simulink model "MPC_adaptive"  (R2020b)
settings: Solver=VariableStepAuto  StartTime=0.0  StopTime=10.0  RelTol=1e-3
values from neighbouring files (symbols this model uses):
  I_mat = [I_xx I_xy I_xz ... (first row only)    [AngularDynamics_VV.m]    (also in angular_tune_test.m; temp.m)
libraries: mpclib x1, cstblocks x1
settings Model: Creator=Jonathan van Zyl  LastModifiedBy=Jonathan van Zyl

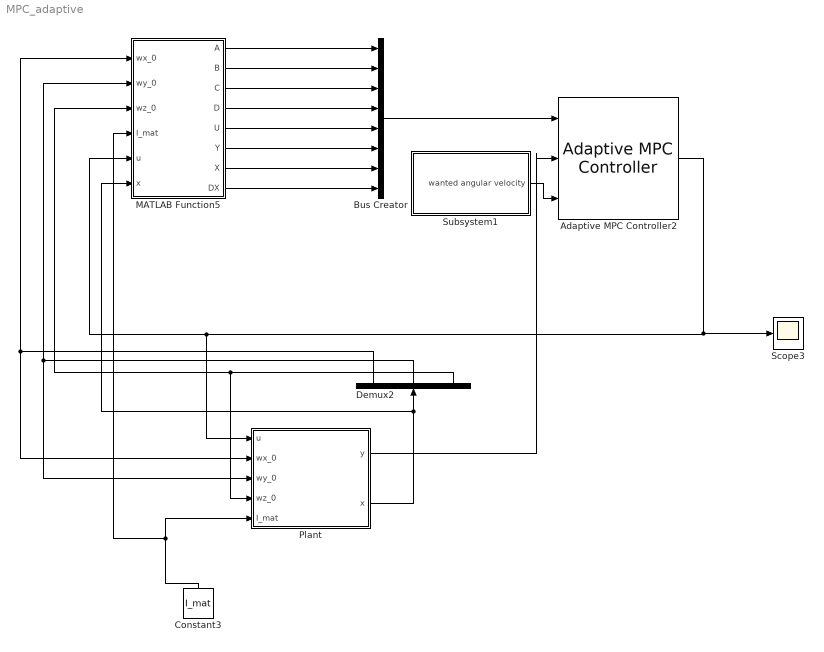
== system MPC_adaptive ==
  Adaptive MPC Controller2 : mpclib/Adaptive MPC Controller  SCDEnableBlockLinearizationSpecification=on  mpcobj=mpc1  enable_value=0  updateMPCinCallerWorkspace=on  md_inport=off  mv_inport=off  uref_inport=off  return_cost=off  return_mvseq=off  return_qpstatus=off  return_xseq=off  return_state=off  return_ovseq=off  state_inport=off  isltv_plant=off  umin_inport=off  umax_inport=off  ymin_inport=off  ymax_inport=off  cc_inport=off  ywt_inport=off  uwt_inport=off  duwt_inport=off  rhoeps_inport=off  pm_inport=off  MaximumP=10  HorizonChoice=FixedHorizon  BlockDataType=double  SampleTimeInherited=off  switch_inport=off
  Bus Creator : BusCreator  Inputs=8
  Constant3 : Constant  Value=I_mat
  Demux2 : Demux  Outputs=3
  MATLAB Function5 : MATLAB Function  TreatAsAtomicUnit=on
  Plant : Subsystem
  Scope3 : Scope
  Subsystem1 : Subsystem
  wires:
  Demux2/2 -> Plant/3(wy_0), MATLAB Function5/2(wy_0)
  Demux2/3 -> MATLAB Function5/3(wz_0), Plant/4(wz_0)
  Constant3/1 -> MATLAB Function5/4(I_mat), Plant/5(I_mat)
  MATLAB Function5/3(C) -> Bus Creator/3
  MATLAB Function5/6(Y) -> Bus Creator/6
  MATLAB Function5/2(B) -> Bus Creator/2
  MATLAB Function5/7(X) -> Bus Creator/7
  MATLAB Function5/8(DX) -> Bus Creator/8
  MATLAB Function5/1(A) -> Bus Creator/1
  MATLAB Function5/4(D) -> Bus Creator/4
  Demux2/1 -> MATLAB Function5/1(wx_0), Plant/2(wx_0)
  MATLAB Function5/5(U) -> Bus Creator/5
  Subsystem1/1(wanted angular velocity) -> Adaptive MPC Controller2/3
  Bus Creator/1 -> Adaptive MPC Controller2/1
  Plant/1(y) -> Adaptive MPC Controller2/2
  Plant/2(x) -> MATLAB Function5/6(x), Demux2/1
  Adaptive MPC Controller2/1 -> MATLAB Function5/5(u), Plant/1(u), Scope3/1

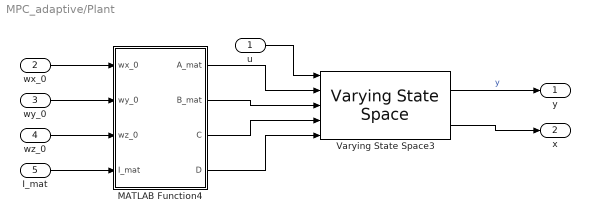
== system MPC_adaptive/Plant ==
  u : Inport
  wx_0 : Inport  Port=2
  wy_0 : Inport  Port=3
  wz_0 : Inport  Port=4
  I_mat : Inport  Port=5
  MATLAB Function4 : MATLAB Function  TreatAsAtomicUnit=on
  Varying State Space3 : cstblocks/Linear Parameter Varying/Varying State Space  x0=[0;0;0]  xNames=''  OutputX=on  OutputDX=off
  y : Outport
  x : Outport  Port=2
  wires:
  MATLAB Function4/4(D) -> Varying State Space3/5
  I_mat/1 -> MATLAB Function4/4(I_mat)
  wy_0/1 -> MATLAB Function4/2(wy_0)
  MATLAB Function4/1(A_mat) -> Varying State Space3/2
  MATLAB Function4/3(C) -> Varying State Space3/4
  wx_0/1 -> MATLAB Function4/1(wx_0)
  MATLAB Function4/2(B_mat) -> Varying State Space3/3
  Varying State Space3/1 -> y/1  "y"
  Varying State Space3/2 -> x/1
  u/1 -> Varying State Space3/1
  wz_0/1 -> MATLAB Function4/3(wz_0)

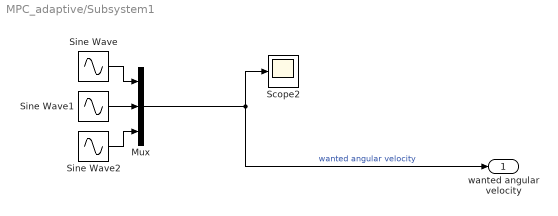
== system MPC_adaptive/Subsystem1 ==
  Mux : Mux  Inputs=3
  Scope2 : Scope
  Sine Wave : Sin  SampleTime=0
  Sine Wave1 : Sin  Amplitude=0.5  Frequency=0.7  SampleTime=0
  Sine Wave2 : Sin  Amplitude=4  Frequency=0.5  SampleTime=0
  wanted angular velocity : Outport
  wires:
  Mux/1 -> wanted angular velocity/1, Scope2/1  "wanted angular velocity"
  Sine Wave2/1 -> Mux/3
  Sine Wave/1 -> Mux/1
  Sine Wave1/1 -> Mux/2

== matlab function MPC_adaptive/Plant/MATLAB Function4 ==
  data: wx_0 input; A_mat output; wy_0 input; wz_0 input; I_mat input; B_mat output; C output; D output
function[A_mat, B_mat, C, D] = func(wx_0, wy_0, wz_0, I_mat)
I_xx = I_mat(1,1);
I_xy = I_mat(1,2);
I_xz = I_mat(1,3);

I_yx = I_mat(2,1);
I_yy = I_mat(2,2);
I_yz = I_mat(2,3);

I_zx = I_mat(3,1);
I_zy = I_mat(3,2);
I_zz = I_mat(3,3);
%% Calculate A matrix
%Calculate numerators
a = (I_yy*I_zz - I_yz*I_zy)*(I_zx*wy_0 - I_yx*wz_0) + (I_xx*I_zy - I_xy*I_zz)*(I_xx*wz_0 - I_zx*wy_0 - I_zz*wz_0) + (I_xy*I_yz - I_xz*I_yy)*(I_zx*wx_0 + I_zy*wy_0 + I_zz*wz_0 - I_yx*wy_0);
b = (I_yy*I_zz - I_yz*I_zy)*(I_zx*wx_0 + I_zy*wy_0 + I_zz*wz_0 - I_yy*wz_0) + (I_xz*I_zy - I_xy*I_zz)*(I_xy*wz_0 - I_zz*wx_0) + (I_xy*I_yz - I_xz*I_yy)*(I_zz*wx_0 - I_yx*wx_0 - I_yy*wy_0 - I_yz*wz_0);
c = (I_yy*I_zz - I_yz*I_zy)*(I_zz*wy_0 - I_yx*wx_0 - I_yy*wy_0 - I_yz*wz_0) + (I_xz*I_zy - I_xy*I_zz)*(I_xx*wx_0 + I_xy*wy_0 + I_xz*wz_0 - I_zz*wx_0) + (I_xy*I_yz - I_xz*I_yy)*(I_zz*wx_0 - I_yz*wy_0);
d = (I_yz*I_zx - I_yx*I_zz)*(I_zx*wy_0 - I_yx*wz_0) + (I_xx*I_zz - I_xz*I_zx)*(I_xx*wz_0 - I_zx*wx_0 - I_zy*wy_0 - I_zz*wz_0) + (I_xz*I_yx - I_xx*I_yz)*(I_zx*wx_0 + I_zz*wz_0 - I_yx*wy_0);
e = (I_yz*I_zx - I_yx*I_zz)*(I_zx*wx_0 + I_zy*wy_0 + I_zz*wz_0 - I_yy*wz_0) + (I_xx*I_zz - I_xz*I_zx)*(I_xy*wz_0 - I_zz*wz_0) + (I_xz*I_yx - I_xx*I_yz)*(I_zz*wx_0 - I_yx*wx_0 - I_yy*wy_0 - I_yz*wz_0);
f = (I_yz*I_zx - I_yx*I_zz)*(I_zz*wy_0 - I_yx*wx_0 - I_yy*wy_0 -I_yz*wz_0) + (I_xx*I_zz - I_xz*I_zx)*(I_xx*wx_0 + I_xy*wy_0 + I_xz*wz_0 - I_zz*wx_0) + (I_xz*I_yx - I_xx*I_yz)*(I_zz*wx_0 - I_yz*wy_0);
g = (I_yx*I_zy - I_yy*I_zx)*(I_zx*wy_0 - I_yx*wz_0) + (I_xy*I_zx - I_xx*I_zy)*(I_xx*wz_0 - I_zx*wx_0 - I_zy*wy_0 - I_zz*wz_0) + (I_xx*I_yy - I_xy*I_yx)*(I_zx*wx_0 + I_zy*wy_0 + I_zz*wz_0 - I_yx*wy_0);
h = (I_yx*I_zy - I_yy*I_zx)*(I_zx*wx_0 + I_zy*wy_0 + I_zz*wz_0 - I_yy*wz_0) + (I_xy*I_zx - I_xx*I_zy)*(I_xy*wz_0 - I_zz*wx_0) + (I_xx*I_yy - I_xy*I_yx)*(I_zz*wx_0 - I_yx*wx_0 - I_yy*wy_0 - I_yz*wz_0);
i = (I_yx*I_zy - I_yy*I_zx)*(I_zz*wy_0 - I_yx*wx_0 - I_yy*wy_0 - I_yz*wz_0) + (I_xy*I_zx - I_xx*I_zy)*(I_xx*wx_0 + I_xy*wy_0 + I_xz*wz_0 - I_zz*wx_0) + (I_xx*I_yy - I_xy*I_yx)*(I_zz*wx_0 - I_yz*wy_0);
%Calculate denominator
A_d= I_xx*I_yy*I_zz + I_xy*I_yz*I_zx + I_xz*I_yx*I_zy - I_zx*I_yy*I_xz - I_zy*I_yz*I_xx - I_zz*I_yx*I_xy;
%Form A-matrix
A_mat = [a/A_d b/A_d c/A_d;
    d/A_d e/A_d f/A_d;
    g h i;];

%% Calculate B-matrix
ab = (I_yy*I_zz - I_yz*I_zy)/A_d;
bb = (I_xz*I_zy - I_xy*I_zz)/A_d;
cb = (I_xy*I_yz - I_xz*I_yy)/A_d;
db = (I_yz*I_zx - I_yx*I_zz)/A_d;
eb = (I_xx*I_zz - I_xz*I_zx)/A_d;
fb = (I_xz*I_yx - I_xx*I_yz)/A_d;
gb = (I_yx*I_zy - I_yy*I_zx)/A_d;
hb = (I_xy*I_zx - I_xx*I_zy)/A_d;
ib = (I_xx*I_yy - I_zy*I_yx)/A_d;

B_mat = [ab bb cb;
    db eb fb;
    gb hb ib;];

%% Make C & D matrix

C = eye(3);
D = zeros(3);
end

== matlab function MPC_adaptive/MATLAB Function5 ==
  data: wx_0 input; A output; wy_0 input; wz_0 input; I_mat input; B output; C output; D output; U output; Y output; X output; DX output; u input; x input
function [A,B,C,D,U,Y,X,DX] = fcn(wx_0, wy_0, wz_0, I_mat, u, x)
% Sample time
Ts = 0.1;

% Model parameters
I_xx = I_mat(1,1);
I_xy = I_mat(1,2);
I_xz = I_mat(1,3);

I_yx = I_mat(2,1);
I_yy = I_mat(2,2);
I_yz = I_mat(2,3);

I_zx = I_mat(3,1);
I_zy = I_mat(3,2);
I_zz = I_mat(3,3);

% Continuous-time model
%Calculate numerators
a = (I_yy*I_zz - I_yz*I_zy)*(I_zx*wy_0 - I_yx*wz_0) + (I_xx*I_zy - I_xy*I_zz)*(I_xx*wz_0 - I_zx*wy_0 - I_zz*wz_0) + (I_xy*I_yz - I_xz*I_yy)*(I_zx*wx_0 + I_zy*wy_0 + I_zz*wz_0 - I_yx*wy_0);
b = (I_yy*I_zz - I_yz*I_zy)*(I_zx*wx_0 + I_zy*wy_0 + I_zz*wz_0 - I_yy*wz_0) + (I_xz*I_zy - I_xy*I_zz)*(I_xy*wz_0 - I_zz*wx_0) + (I_xy*I_yz - I_xz*I_yy)*(I_zz*wx_0 - I_yx*wx_0 - I_yy*wy_0 - I_yz*wz_0);
c = (I_yy*I_zz - I_yz*I_zy)*(I_zz*wy_0 - I_yx*wx_0 - I_yy*wy_0 - I_yz*wz_0) + (I_xz*I_zy - I_xy*I_zz)*(I_xx*wx_0 + I_xy*wy_0 + I_xz*wz_0 - I_zz*wx_0) + (I_xy*I_yz - I_xz*I_yy)*(I_zz*wx_0 - I_yz*wy_0);
d = (I_yz*I_zx - I_yx*I_zz)*(I_zx*wy_0 - I_yx*wz_0) + (I_xx*I_zz - I_xz*I_zx)*(I_xx*wz_0 - I_zx*wx_0 - I_zy*wy_0 - I_zz*wz_0) + (I_xz*I_yx - I_xx*I_yz)*(I_zx*wx_0 + I_zz*wz_0 - I_yx*wy_0);
e = (I_yz*I_zx - I_yx*I_zz)*(I_zx*wx_0 + I_zy*wy_0 + I_zz*wz_0 - I_yy*wz_0) + (I_xx*I_zz - I_xz*I_zx)*(I_xy*wz_0 - I_zz*wz_0) + (I_xz*I_yx - I_xx*I_yz)*(I_zz*wx_0 - I_yx*wx_0 - I_yy*wy_0 - I_yz*wz_0);
f = (I_yz*I_zx - I_yx*I_zz)*(I_zz*wy_0 - I_yx*wx_0 - I_yy*wy_0 -I_yz*wz_0) + (I_xx*I_zz - I_xz*I_zx)*(I_xx*wx_0 + I_xy*wy_0 + I_xz*wz_0 - I_zz*wx_0) + (I_xz*I_yx - I_xx*I_yz)*(I_zz*wx_0 - I_yz*wy_0);
g = (I_yx*I_zy - I_yy*I_zx)*(I_zx*wy_0 - I_yx*wz_0) + (I_xy*I_zx - I_xx*I_zy)*(I_xx*wz_0 - I_zx*wx_0 - I_zy*wy_0 - I_zz*wz_0) + (I_xx*I_yy - I_xy*I_yx)*(I_zx*wx_0 + I_zy*wy_0 + I_zz*wz_0 - I_yx*wy_0);
h = (I_yx*I_zy - I_yy*I_zx)*(I_zx*wx_0 + I_zy*wy_0 + I_zz*wz_0 - I_yy*wz_0) + (I_xy*I_zx - I_xx*I_zy)*(I_xy*wz_0 - I_zz*wx_0) + (I_xx*I_yy - I_xy*I_yx)*(I_zz*wx_0 - I_yx*wx_0 - I_yy*wy_0 - I_yz*wz_0);
i = (I_yx*I_zy - I_yy*I_zx)*(I_zz*wy_0 - I_yx*wx_0 - I_yy*wy_0 - I_yz*wz_0) + (I_xy*I_zx - I_xx*I_zy)*(I_xx*wx_0 + I_xy*wy_0 + I_xz*wz_0 - I_zz*wx_0) + (I_xx*I_yy - I_xy*I_yx)*(I_zz*wx_0 - I_yz*wy_0);
%Calculate denominator
A_d= I_xx*I_yy*I_zz + I_xy*I_yz*I_zx + I_xz*I_yx*I_zy - I_zx*I_yy*I_xz - I_zy*I_yz*I_xx - I_zz*I_yx*I_xy;
%Form A-matrix
Ac = [a/A_d b/A_d c/A_d;
    d/A_d e/A_d f/A_d;
    g h i;];

ab = (I_yy*I_zz - I_yz*I_zy)/A_d;
bb = (I_xz*I_zy - I_xy*I_zz)/A_d;
cb = (I_xy*I_yz - I_xz*I_yy)/A_d;
db = (I_yz*I_zx - I_yx*I_zz)/A_d;
eb = (I_xx*I_zz - I_xz*I_zx)/A_d;
fb = (I_xz*I_yx - I_xx*I_yz)/A_d;
gb = (I_yx*I_zy - I_yy*I_zx)/A_d;
hb = (I_xy*I_zx - I_xx*I_zy)/A_d;
ib = (I_xx*I_yy - I_zy*I_yx)/A_d;

Bc = [ab bb cb;
    db eb fb;
    gb hb ib;];

Cc = eye(3);
Dc = zeros(3);

% Generate discrete-time model
nx = size(Ac,1);
nu = size(Bc,2);
M = expm([[Ac Bc]*Ts; zeros(nu,nx+nu)]);
A = M(1:nx,1:nx);
B = M(1:nx,nx+1:nx+nu);
C = Cc;
D = Dc;

% Nominal conditions for discrete-time plant
X = x;
U = u;
Y = C*x + D*u;
DX = A*x+B*u-x;
end
